simulink model "ODE6"  (Simulink 7.8)
settings: Solver=ode4  StartTime=0.0  StopTime=time_span  RelTol=1e-3
undefined symbols (not defined in the file): samp_time, x
settings Model: Creator=Kourosh Danai  LastModifiedBy=BionicBill
settings DebuggingCC: AlgebraicLoopMsg=none  SolverPrmCheckMsg=none  FcnCallInpInsideContextMsg=Use local settings  StrictBusMsg=Warning
settings SFSimCC: SimParseCustomCode=off

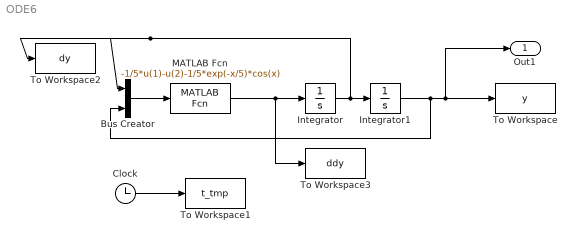
== system ODE6 ==
  Bus Creator : BusCreator  Inputs=2
  Clock : Clock
  Integrator : Integrator  InitialCondition=1
  Integrator1 : Integrator
  MATLAB Fcn : MATLABFcn  MATLABFcn=-1/5*u(1)-u(2)-1/5*exp(-x/5)*cos(x)  SampleTime=samp_time
  To Workspace : ToWorkspace  VariableName=y  SampleTime=-1  SaveFormat=Array
  To Workspace1 : ToWorkspace  VariableName=t_tmp  SampleTime=-1  SaveFormat=Array
  To Workspace2 : ToWorkspace  VariableName=dy  SampleTime=-1  SaveFormat=Array
  To Workspace3 : ToWorkspace  VariableName=ddy  SampleTime=-1  SaveFormat=Array
  Out1 : Outport
  wires:
  Integrator/1 -> Integrator1/1, Bus Creator/1, To Workspace2/1
  Bus Creator/1 -> MATLAB Fcn/1
  Clock/1 -> To Workspace1/1
  Integrator1/1 -> To Workspace/1, Out1/1, Bus Creator/2
  MATLAB Fcn/1 -> Integrator/1, To Workspace3/1
